simulink model "PWM_Conversion_MATLABFunction_block"  (R2019b)
settings: Solver=VariableStepAuto  StartTime=0.0  StopTime=10.0  RelTol=1e-3
settings Model: Creator=spuny  LastModifiedBy=spuny

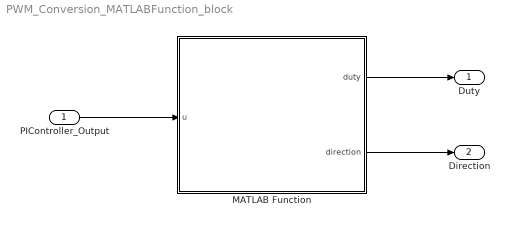
== system PWM_Conversion_MATLABFunction_block ==
  "PIController_Output " : Inport
  MATLAB Function : MATLAB Function  TreatAsAtomicUnit=on
  Duty : Outport
  "Direction " : Outport  Port=2
  wires:
  MATLAB Function/1(duty) -> Duty/1
  MATLAB Function/2(direction) -> "Direction "/1
  "PIController_Output "/1 -> MATLAB Function/1(u)

== matlab function PWM_Conversion_MATLABFunction_block/MATLAB Function ==
  data: u input; duty output; direction output
function [duty,direction]=u2dd(u)

%Set direction bit and set duty = abd(u)

if u>= 0
    duty = u;
    direction = 1;
else
    duty = -u;
    direction=-1;
end
%Saturate duty cycle to 1

if duty>1
    duty =1;
end
